simulink model "mass_spring_dampersystem"  (R2018a)
settings: Solver=VariableStepAuto  StartTime=0.0  StopTime=sim_Time  RelTol=1e-3
values from neighbouring files (symbols this model uses):
  b = 1    [mass_spring_value.m]
  F = 1    [mass_spring_value.m]
  k = 20    [mass_spring_value.m]
  M = 1    [mass_spring_value.m]
settings Model: Creator=Keshav Mishra  LastModifiedBy=Keshav Mishra

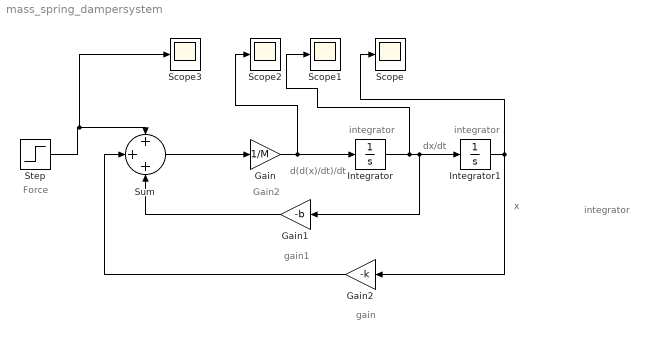
== system mass_spring_dampersystem ==
  note: x
  note: dx/dt
  note: d(d(x)/dt)/dt
  note: integrator
  note: integrator
  note: gain
  note: gain1
  note: Gain2
  note: Force
  note: integrator
  Gain : Gain  Gain=1/M
  Gain1 : Gain  Gain=-b
  Gain2 : Gain  Gain=-k
  Integrator : Integrator
  Integrator1 : Integrator
  Scope{,1..3} (4 alike) : Scope
  Step : Step  After=F  SampleTime=0
  Sum : Sum  Inputs=+++
  wires:
  Step/1 -> Scope3/1, Sum/1
  Sum/1 -> Gain/1
  Gain/1 -> Integrator/1, Scope2/1
  Integrator/1 -> Scope1/1, Gain1/1, Integrator1/1
  Integrator1/1 -> Scope/1, Gain2/1
  Gain1/1 -> Sum/3
  Gain2/1 -> Sum/2
